simulink model "pendule_inv_echant_etu"  (R2021a)
settings: Solver=VariableStepAuto  StartTime=0.0  StopTime=10.0  RelTol=1e-3
values from neighbouring files (symbols this model uses):
  delta_t = 0.4    [simu_pendule_inv_echant_etu.m]
  g = 9.81    [simu_pendule_inv_capteur_etu.m]    (also in simu_pendule_inv_echant_etu.m; simu_pendule_inv_etu.m)
  K = [10 1]    [simu_pendule_inv_capteur_etu.m]    (also in simu_pendule_inv_echant_etu.m = [30 10]; simu_pendule_inv_etu.m = [30 10])
  l = 10    [simu_pendule_inv_capteur_etu.m]    (also in simu_pendule_inv_echant_etu.m; simu_pendule_inv_etu.m)
  ue = 0    [simu_pendule_inv_capteur_etu.m]    (also in simu_pendule_inv_echant_etu.m; simu_pendule_inv_etu.m)
  x0 = [pi/20 0]'    [simu_pendule_inv_capteur_etu.m]    (also in simu_pendule_inv_echant_etu.m; simu_pendule_inv_etu.m = [pi/10 0])
  xe = [0 0]'    [simu_pendule_inv_capteur_etu.m]    (also in simu_pendule_inv_echant_etu.m; simu_pendule_inv_etu.m)
undefined symbols (not defined in the file or in its folder): DiscIntNeverNeededParam
settings Model: Creator=aseghrou  LastModifiedBy=aseghrou

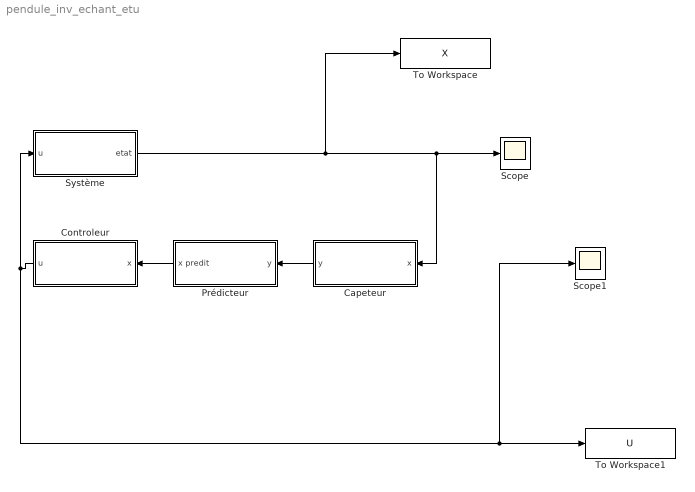
== system pendule_inv_echant_etu ==
  Capeteur : Subsystem
  Controleur : Subsystem
  Prédicteur : Subsystem
  Scope : Scope
  Scope1 : Scope
  Système : Subsystem
  To Workspace : ToWorkspace  VariableName=X  SaveFormat=Timeseries  SampleTime=-1
  To Workspace1 : ToWorkspace  VariableName=U  SaveFormat=Timeseries  SampleTime=-1
  wires:
  Système/1(etat) -> To Workspace/1, Capeteur/1(x), Scope/1
  Capeteur/1(y) -> Prédicteur/1(y)
  Prédicteur/1(x predit) -> Controleur/1(x)
  Controleur/1(u) -> Système/1(u), Scope1/1, To Workspace1/1

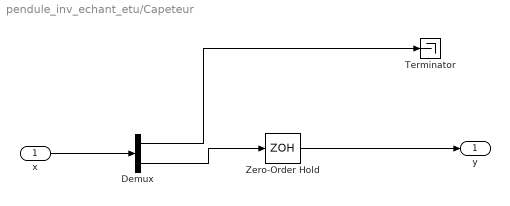
== system pendule_inv_echant_etu/Capeteur ==
  x : Inport
  Demux : Demux  Outputs=2
  Terminator : Terminator
  Zero-Order Hold : ZeroOrderHold  SampleTime=delta_t
  y : Outport
  wires:
  x/1 -> Demux/1
  Demux/2 -> Zero-Order Hold/1
  Zero-Order Hold/1 -> y/1
  Demux/1 -> Terminator/1

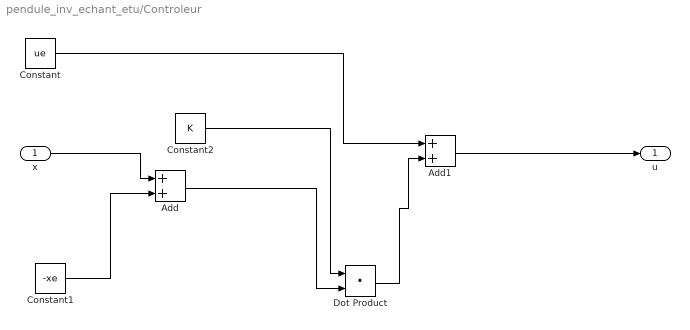
== system pendule_inv_echant_etu/Controleur ==
  x : Inport
  Add : Sum
  Add1 : Sum
  Constant : Constant  Value=ue
  Constant1 : Constant  Value=-xe
  Constant2 : Constant  Value=K
  Dot Product : DotProduct  InputSameDT=on  OutDataTypeStr=Inherit: Inherit via internal rule
  u : Outport
  wires:
  x/1 -> Add/1
  Add1/1 -> u/1
  Constant1/1 -> Add/2
  Add/1 -> Dot Product/2
  Constant2/1 -> Dot Product/1
  Constant/1 -> Add1/1
  Dot Product/1 -> Add1/2

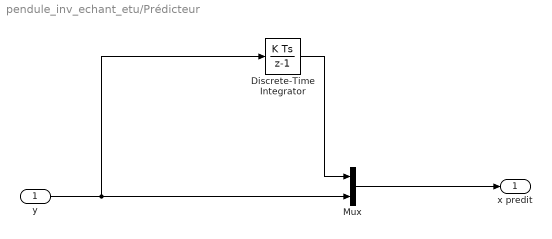
== system pendule_inv_echant_etu/Prédicteur ==
  y : Inport
  Discrete-Time Integrator : DiscreteIntegrator  InitialCondition=x0(1)  SampleTime=delta_t  ICPrevOutput=DiscIntNeverNeededParam  ICPrevScaledInput=DiscIntNeverNeededParam
  Mux : Mux  Inputs=2
  x predit : Outport
  wires:
  y/1 -> Discrete-Time Integrator/1, Mux/2
  Discrete-Time Integrator/1 -> Mux/1
  Mux/1 -> x predit/1

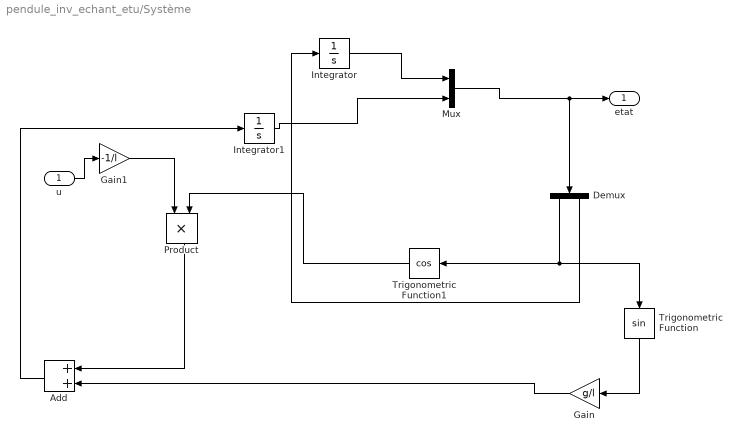
== system pendule_inv_echant_etu/Système ==
  u : Inport
  Add : Sum
  Demux : Demux  Outputs=2
  Gain : Gain  Gain=g/l
  Gain1 : Gain  Gain=-1/l
  Integrator : Integrator  InitialCondition=x0(1)
  Integrator1 : Integrator  InitialCondition=x0(2)
  Mux : Mux  Inputs=2
  Product : Product
  Trigonometric Function : Trigonometry
  Trigonometric Function1 : Trigonometry  Operator=cos
  etat : Outport
  wires:
  Mux/1 -> Demux/1, etat/1
  Demux/1 -> Trigonometric Function/1, Trigonometric Function1/1
  Trigonometric Function/1 -> Gain/1
  Gain/1 -> Add/2
  u/1 -> Gain1/1
  Gain1/1 -> Product/1
  Trigonometric Function1/1 -> Product/2
  Product/1 -> Add/1
  Add/1 -> Integrator1/1
  Integrator1/1 -> Mux/2
  Integrator/1 -> Mux/1
  Demux/2 -> Integrator/1
